simulink model "ControleLQRTrajNominalSimulink"  (R2019a)
settings: Solver=VariableStepAuto  StartTime=0.0  StopTime=170  RelTol=1e-3
undefined symbols (not defined in the file): A, B, K
settings Model: Creator=Cliente  LastModifiedBy=Cliente

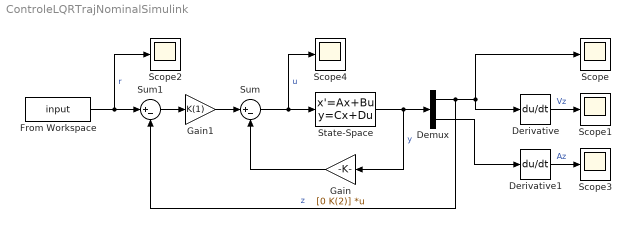
== system ControleLQRTrajNominalSimulink ==
  Demux : Demux  Outputs=2
  Derivative : Derivative
  Derivative1 : Derivative
  From Workspace : FromWorkspace  VariableName=input  SampleTime=0
  Gain : Gain  Gain=[0 K(2)]  Multiplication=Matrix(K*u) (u vector)
  Gain1 : Gain  Gain=K(1)
  Scope{,1..4} (5 alike) : Scope
  State-Space : StateSpace  A=A  B=B  C=[1 0;0 1]  D=[0;0]  InitialCondition=[0; 0]
  Sum : Sum  Inputs=|+-
  Sum1 : Sum  Inputs=|+-
  wires:
  State-Space/1 -> Demux/1, Gain/1  "y"
  Demux/2 -> Derivative1/1
  Sum/1 -> State-Space/1, Scope4/1  "u"
  Gain/1 -> Sum/2
  Derivative1/1 -> Scope3/1  "Az"
  Demux/1 -> Scope/1, Derivative/1, Sum1/2  "z"
  Derivative/1 -> Scope1/1  "Vz"
  From Workspace/1 -> Scope2/1, Sum1/1  "r"
  Gain1/1 -> Sum/1
  Sum1/1 -> Gain1/1
